simulink model "Final_Longitudinal"  (R2021a)
settings: Solver=VariableStepAuto  StartTime=0.0  StopTime=20  MinStep=0.001  RelTol=1e-6  AbsTol=1e-6
undefined symbols (not defined in the file or in its folder): AL, BL, KL, kli
libraries: dspsrcs4 x1
settings Model: Creator=Lenovo  LastModifiedBy=Lenovo
settings SolverCC: InitialStep=0.01

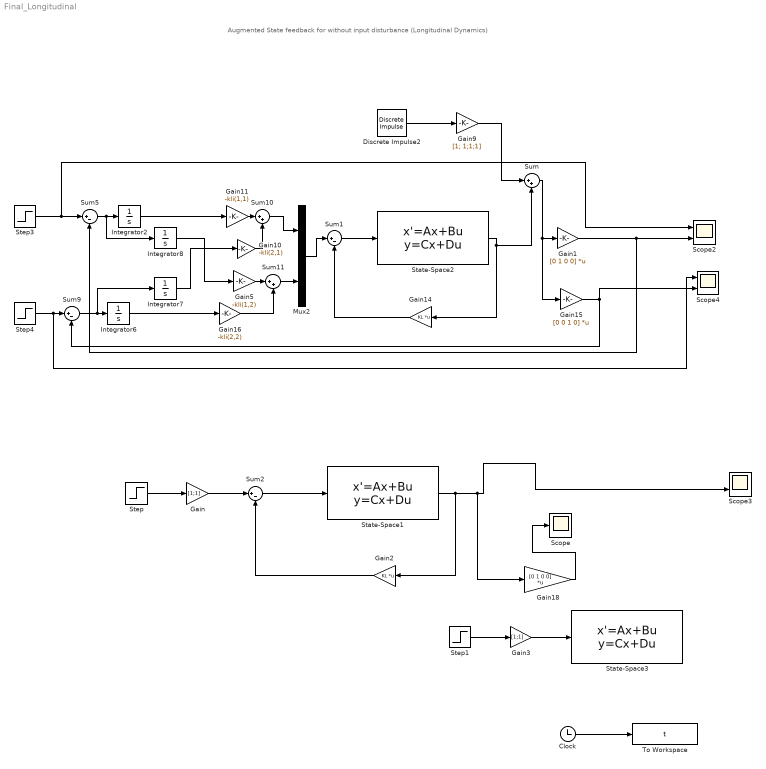
== system Final_Longitudinal ==
  note: Augmented State feedback for without input disturbance (Longitudinal Dynamics)
  Clock : Clock
  Discrete Impulse2 : dspsrcs4/Discrete  Impulse  Delay=0  SampleTime=1  FrameSample=1  OutputFrames=off  dataType=double  isSigned=on  wordLen=16  udDataType=sfix(16)  fracBitsMode=Best precision  numFracBits=15  OutDataTypeStr=double  LastOutDataTypeStr=double
  Gain : Gain  Gain=[1;1]
  Gain1 : Gain  Gain=[0 1 0 0]  Multiplication=Matrix(K*u) (u vector)
  Gain10 : Gain  Gain=-kli(2,1)
  Gain11 : Gain  Gain=-kli(1,1)
  Gain14 : Gain  Gain=KL  Multiplication=Matrix(K*u)
  Gain15 : Gain  Gain=[0 0 1 0]  Multiplication=Matrix(K*u) (u vector)
  Gain16 : Gain  Gain=-kli(2,2)
  Gain18 : Gain  Gain=[0 1 0 0]  Multiplication=Matrix(K*u)
  Gain2 : Gain  Gain=KL  Multiplication=Matrix(K*u)
  Gain3 : Gain  Gain=[1;1]
  Gain5 : Gain  Gain=-kli(1,2)
  Gain9 : Gain  Gain=[1; 1;1;1]
  Integrator{2,6..8} (4 alike) : Integrator
  Mux2 : Mux  Inputs=2
  Scope : Scope
  Scope2 : Scope  NumInputPorts=2
  Scope3 : Scope  NumInputPorts=2
  Scope4 : Scope  NumInputPorts=2
  State-Space1 : StateSpace  A=AL  B=BL  C=[0 0 0 0; 0 1 0 0; 0 0 1 0; 0 0 0 0]  D=zeros(4,2)  InitialCondition=0
  State-Space2 : StateSpace  A=AL  B=BL  C=eye(4)  D=zeros(4,2)  InitialCondition=0
  State-Space3 : StateSpace  A=AL  B=BL  C=[0 0 0 0; 0 1 0 0; 0 0 1 0; 0 0 0 0]  D=zeros(4,2)  InitialCondition=0
  Step{,1,3..4} (4 alike) : Step  Time=0  SampleTime=0
  Sum : Sum  Inputs=|++
  Sum{1..2,5,9} (4 alike) : Sum  Inputs=|+-
  Sum10 : Sum  Inputs=|++
  Sum11 : Sum  Inputs=|++
  To Workspace : ToWorkspace  VariableName=t
  wires:
  Gain16/1 -> Sum11/2
  Gain14/1 -> Sum1/2
  Sum10/1 -> Mux2/1
  Gain15/1 -> Scope4/2, Sum9/2
  Gain5/1 -> Sum11/1
  Integrator2/1 -> Gain11/1
  Integrator7/1 -> Gain10/1
  Gain10/1 -> Sum10/2
  Gain11/1 -> Sum10/1
  Sum11/1 -> Mux2/2
  Gain1/1 -> Scope2/2, Sum5/2
  Integrator8/1 -> Gain5/1
  Integrator6/1 -> Gain16/1
  Sum1/1 -> State-Space2/1
  Step4/1 -> Scope4/1, Sum9/1
  Step3/1 -> Sum5/1, Scope2/1
  Sum5/1 -> Integrator8/1, Integrator2/1
  Mux2/1 -> Sum1/1
  Sum9/1 -> Integrator7/1, Integrator6/1
  Sum2/1 -> State-Space1/1
  Gain2/1 -> Sum2/2
  State-Space1/1 -> Gain2/1, Gain18/1, Scope3/2
  Step/1 -> Gain/1
  Gain/1 -> Sum2/1
  Gain3/1 -> State-Space3/1
  Step1/1 -> Gain3/1
  Discrete Impulse2/1 -> Gain9/1
  State-Space2/1 -> Sum/2, Gain14/1
  Clock/1 -> To Workspace/1
  Gain18/1 -> Scope/1
  Gain9/1 -> Sum/1
  Sum/1 -> Gain1/1, Gain15/1
